simulink model "L9_tank_PID"  (R2015b)
settings: Solver=VariableStepAuto  StartTime=0.0  StopTime=300  RelTol=1e-3
undefined symbols (not defined in the file or in its folder): G_PID_PAR, tank_pid
settings Model: Creator=kjartan  LastModifiedBy=kjartan

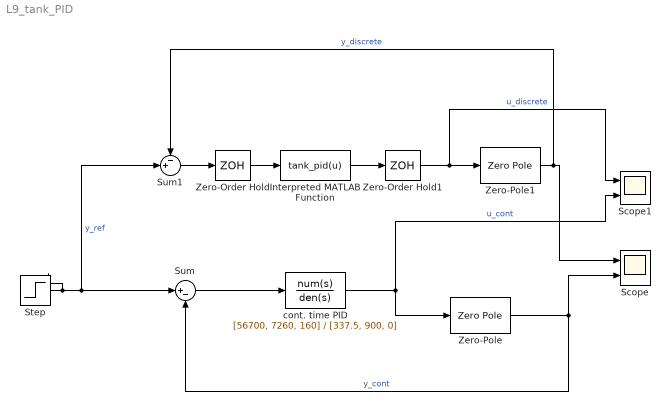
== system L9_tank_PID ==
  Interpreted MATLAB Function : MATLABFcn  MATLABFcn=tank_pid(u)  OutputDimensions=1
  Scope : Scope  NumInputPorts=2
  Scope1 : Scope  NumInputPorts=2
  Step : Step  SampleTime=0
  Sum : Sum  Inputs=|+-
  Sum1 : Sum  Inputs=-+|
  Zero-Order Hold : ZeroOrderHold  SampleTime=G_PID_PAR.h
  Zero-Order Hold1 : ZeroOrderHold  SampleTime=G_PID_PAR.h
  Zero-Pole : ZeroPole  Zeros=[]  Poles=[-0.0179, -0.0129]  Gain=[0.00048]
  Zero-Pole1 : ZeroPole  Zeros=[]  Poles=[-0.0179, -0.0129]  Gain=[0.00048]
  cont. time PID : TransferFcn  Numerator=[56700, 7260, 160]  Denominator=[337.5, 900, 0]
  wires:
  Sum/1 -> cont. time PID/1
  Zero-Pole/1 -> Scope/2, Sum/2  "y_cont"
  Step/1 -> Sum1/2, Sum/1  "y_ref"
  Zero-Order Hold/1 -> Interpreted MATLAB Function/1
  Interpreted MATLAB Function/1 -> Zero-Order Hold1/1
  Zero-Order Hold1/1 -> Scope1/1, Zero-Pole1/1  "u_discrete"
  cont. time PID/1 -> Scope1/2, Zero-Pole/1  "u_cont"
  Zero-Pole1/1 -> Scope/1, Sum1/1  "y_discrete"
  Sum1/1 -> Zero-Order Hold/1
